simulink model "stm32f4_ds3231_configure_demo"  (Simulink 7.3)
settings: Solver=FixedStepDiscrete  SolverMode=SingleTasking  StartTime=0.0  StopTime=10.0  RelTol=1e-3
PreLoadFcn:
  | waijung.modelPreload; % Required for working with Waijung Blockset. Do not remove.
undefined symbols (not defined in the file): HSEOSC, Link, LQFP176, ST, STM32F417IG
libraries: simulink x94, amg_high_precision_rtc x5, stm32f4_io_lib x2, stm32f4_device_config_lib x1
(part 4 of 4)

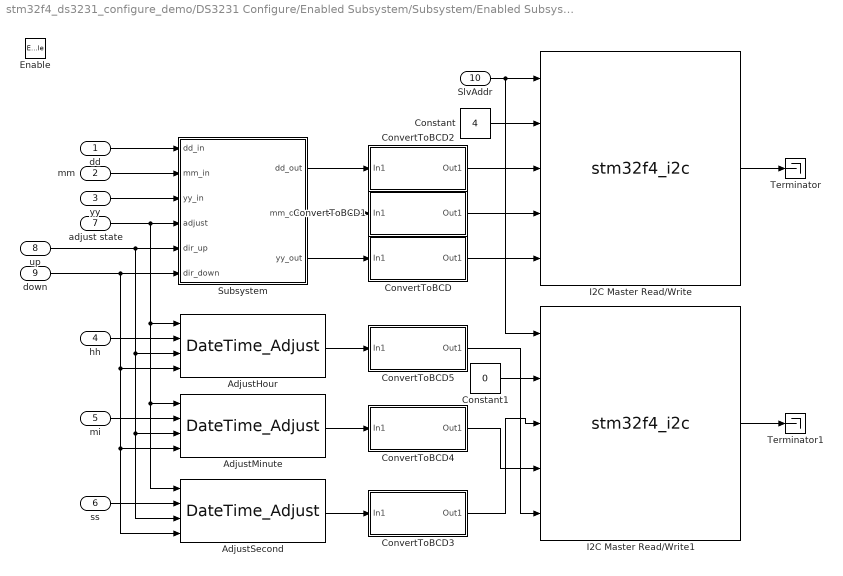
== system stm32f4_ds3231_configure_demo/DS3231 Configure/Enabled Subsystem/Subsystem/Enabled Subsystem ==
  dd : Inport  OutDataType=fixdt(1, 16)  OutScaling=2^0
  mm : Inport  Port=2  OutDataType=fixdt(1, 16)  OutScaling=2^0
  yy : Inport  Port=3  OutDataType=fixdt(1, 16)  OutScaling=2^0
  hh : Inport  Port=4  OutDataType=fixdt(1, 16)  OutScaling=2^0
  mi : Inport  Port=5  OutDataType=fixdt(1, 16)  OutScaling=2^0
  ss : Inport  Port=6  OutDataType=fixdt(1, 16)  OutScaling=2^0
  adjust state : Inport  Port=7  OutDataType=fixdt(1, 16)  OutScaling=2^0
  up : Inport  Port=8  OutDataType=fixdt(1, 16)  OutScaling=2^0
  down : Inport  Port=9  OutDataType=fixdt(1, 16)  OutScaling=2^0
  SlvAddr : Inport  Port=10  OutDataType=fixdt(1, 16)  OutScaling=2^0
  Enable : EnablePort
  AdjustHour : amg_high_precision_rtc/DateTime_Adjust  SystemSampleTime=-1  state=3  max=23  min=0
  AdjustMinute : amg_high_precision_rtc/DateTime_Adjust  SystemSampleTime=-1  state=4  max=59  min=0
  AdjustSecond : amg_high_precision_rtc/DateTime_Adjust  SystemSampleTime=-1  state=5  max=59  min=0
  Constant : Constant  Value=4  OutDataTypeMode=uint8  OutDataType=fixdt(1, 16)  OutScaling=2^0  OutDataTypeStr=uint8
  Constant1 : Constant  Value=0  OutDataTypeMode=uint8  OutDataType=fixdt(1, 16)  OutScaling=2^0  OutDataTypeStr=uint8
  ConvertToBCD : Subsystem  TreatAsAtomicUnit=on
      settings: RTWFcnNameOpts=Use subsystem name  RTWFileNameOpts=Use function name
      mask Display: disp('Dec-to-BCD');
  ConvertToBCD1 : Subsystem  TreatAsAtomicUnit=on
      settings: RTWFcnNameOpts=Use subsystem name  RTWFileNameOpts=Use function name
      mask Display: disp('Dec-to-BCD');
  ConvertToBCD2 : Subsystem  TreatAsAtomicUnit=on
      settings: RTWFcnNameOpts=Use subsystem name  RTWFileNameOpts=Use function name
      mask Display: disp('Dec-to-BCD');
  ConvertToBCD3 : Subsystem  TreatAsAtomicUnit=on
      settings: RTWFcnNameOpts=Use subsystem name  RTWFileNameOpts=Use function name
      mask Display: disp('Dec-to-BCD');
  ConvertToBCD4 : Subsystem  TreatAsAtomicUnit=on
      settings: RTWFcnNameOpts=Use subsystem name  RTWFileNameOpts=Use function name
      mask Display: disp('Dec-to-BCD');
  ConvertToBCD5 : Subsystem  TreatAsAtomicUnit=on
      settings: RTWFcnNameOpts=Use subsystem name  RTWFileNameOpts=Use function name
      mask Display: disp('Dec-to-BCD');
  I2C Master Read/Write : S-Function  FunctionName=stm32f4_i2c  Parameters=configuration,module,transfer,clkspeed,timeout,sdapin,sclpin,writecount,readcount,inputtypearray,outputtypearray,confstr,sampletime,sampletimestr,blockid  EnableBusSupport=off  mask(stm32f4_i2c){configuration=Transaction, module=1, lastmodule=3, transfer=Blocking, dutycycle=TLow/THigh = 2, clkspeed=400, timeout=25, writecount=4, readcount=0, sdapin=C9, sclpin=A8, waitwritetime=0, inputtypearray=[5 3 3 3 3 3], outputtypearray=[1 3], confstr=["C","9","A","8","1","1","6","0","I2C_DutyCycle_2","0","off"], sampletime=-1, sampletimestr=0.01, blockid=DS3231ConfigureEnabledSubsystemSubsystemEnabledSubsystemI2CMasterReadWrite}
      mask prompts: module "I2C Module"; lastmodule "Last module"; transfer "Transfer mode"; dutycycle "Duty cycle in fast mode"; clkspeed "Clock speed (kHz)"; timeout "Timeout (ms)"; writecount "Bytes write count"; readcount "Bytes read count"; sdapin "SDA pin"; sclpin "SCL pin"; waitwritetime "Wait write time (ms), default is 0"; inputtypearray "Input type array"; outputtypearray "Output type array"; confstr "Configuration string"; sampletime "Sample time (sec)"; sampletimestr "Compiled sample time (sec) in string"
      mask init:
      | stm32f4_i2c_callback('init');
      mask Help: web(fullfile(waijungdocroot,'stm32f4_i2c_readwrite.htm'), '-browser')
      mask StyleString: popup(Setup|Transaction),popup(1|2|3),edit,popup(Blocking|Non-blocking),popup(TLow/THigh = 16/9|TLow/THigh = 2),edit,edit,edit,edit,popup(-|C9),popup(-|A8),edit,edit,edit,edit,edit,edit,edit
      mask CallbackString: stm32f4_i2c_callback('configuration');|stm32f4_i2c_callback('module');|||stm32f4_i2c_callback('dutycycle');|||stm32f4_i2c_callback('writecount');|stm32f4_i2c_callback('readcount');|stm32f4_i2c_callback('sdapin');|stm32f4_i2c_callback('sclpin');||||stm32f4_i2c_callback('confstr');|stm32f4_i2c_callback('sampletime');|stm32f4_i2c_callback('sampletimestr');|stm32f4_i2c_callback('blockid');
      mask Display: text(0.5, 0.5, 'Module: I2C1\nTransfer: Blocking\nWrite: 4 bytes\nRead: 0 bytes\nTs (sec): 0.01','ver','middle','hor','center');port_label('input', 1,'SlvAddr');port_label('input', 2,'Wr0 (uint8)');port_label('input', 3,'Wr1 (uint8)');port_label('input', 4,'Wr2 (uint8)');port_label('input', 5,'Wr3 (uint8)');port_label('output', 1,'Status');
  I2C Master Read/Write1 : S-Function  FunctionName=stm32f4_i2c  Parameters=configuration,module,transfer,clkspeed,timeout,sdapin,sclpin,writecount,readcount,inputtypearray,outputtypearray,confstr,sampletime,sampletimestr,blockid  EnableBusSupport=off  mask(stm32f4_i2c){configuration=Transaction, module=1, lastmodule=3, transfer=Blocking, dutycycle=TLow/THigh = 2, clkspeed=400, timeout=25, writecount=4, readcount=0, sdapin=C9, sclpin=A8, waitwritetime=0, inputtypearray=[5 3 3 3 3 3], outputtypearray=[1 3], confstr=["C","9","A","8","1","1","6","0","I2C_DutyCycle_2","0","off"], sampletime=-1, sampletimestr=0.01, blockid=DS3231ConfigureEnabledSubsystemSubsystemEnabledSubsystemI2CMasterReadWrite1}
      mask prompts: module "I2C Module"; lastmodule "Last module"; transfer "Transfer mode"; dutycycle "Duty cycle in fast mode"; clkspeed "Clock speed (kHz)"; timeout "Timeout (ms)"; writecount "Bytes write count"; readcount "Bytes read count"; sdapin "SDA pin"; sclpin "SCL pin"; waitwritetime "Wait write time (ms), default is 0"; inputtypearray "Input type array"; outputtypearray "Output type array"; confstr "Configuration string"; sampletime "Sample time (sec)"; sampletimestr "Compiled sample time (sec) in string"
      mask init:
      | stm32f4_i2c_callback('init');
      mask Help: web(fullfile(waijungdocroot,'stm32f4_i2c_readwrite.htm'), '-browser')
      mask StyleString: popup(Setup|Transaction),popup(1|2|3),edit,popup(Blocking|Non-blocking),popup(TLow/THigh = 16/9|TLow/THigh = 2),edit,edit,edit,edit,popup(-|C9),popup(-|A8),edit,edit,edit,edit,edit,edit,edit
      mask CallbackString: stm32f4_i2c_callback('configuration');|stm32f4_i2c_callback('module');|||stm32f4_i2c_callback('dutycycle');|||stm32f4_i2c_callback('writecount');|stm32f4_i2c_callback('readcount');|stm32f4_i2c_callback('sdapin');|stm32f4_i2c_callback('sclpin');||||stm32f4_i2c_callback('confstr');|stm32f4_i2c_callback('sampletime');|stm32f4_i2c_callback('sampletimestr');|stm32f4_i2c_callback('blockid');
      mask Display: text(0.5, 0.5, 'Module: I2C1\nTransfer: Blocking\nWrite: 4 bytes\nRead: 0 bytes\nTs (sec): 0.01','ver','middle','hor','center');port_label('input', 1,'SlvAddr');port_label('input', 2,'Wr0 (uint8)');port_label('input', 3,'Wr1 (uint8)');port_label('input', 4,'Wr2 (uint8)');port_label('input', 5,'Wr3 (uint8)');port_label('output', 1,'Status');
  Subsystem : Subsystem
  Terminator : Terminator
  Terminator1 : Terminator
  wires:
  ConvertToBCD3/1(Out1) -> I2C Master Read/Write1/3
  ConvertToBCD5/1(Out1) -> I2C Master Read/Write1/5
  AdjustSecond/1 -> ConvertToBCD3/1(In1)
  AdjustMinute/1 -> ConvertToBCD4/1(In1)
  AdjustHour/1 -> ConvertToBCD5/1(In1)
  ConvertToBCD4/1(Out1) -> I2C Master Read/Write1/4
  I2C Master Read/Write1/1 -> Terminator1/1
  Constant1/1 -> I2C Master Read/Write1/2
  hh/1 -> AdjustHour/2
  mi/1 -> AdjustMinute/2
  ss/1 -> AdjustSecond/2
  ConvertToBCD/1(Out1) -> I2C Master Read/Write/5
  ConvertToBCD1/1(Out1) -> I2C Master Read/Write/4
  ConvertToBCD2/1(Out1) -> I2C Master Read/Write/3
  I2C Master Read/Write/1 -> Terminator/1
  Constant/1 -> I2C Master Read/Write/2
  Subsystem/3(yy_out) -> ConvertToBCD/1(In1)
  Subsystem/2(mm_out) -> ConvertToBCD1/1(In1)
  Subsystem/1(dd_out) -> ConvertToBCD2/1(In1)
  SlvAddr/1 -> I2C Master Read/Write1/1, I2C Master Read/Write/1
  down/1 -> AdjustSecond/4, AdjustMinute/4, AdjustHour/4, Subsystem/6(dir_down)
  up/1 -> AdjustSecond/3, AdjustMinute/3, AdjustHour/3, Subsystem/5(dir_up)
  adjust state/1 -> AdjustSecond/1, AdjustMinute/1, AdjustHour/1, Subsystem/4(adjust)
  yy/1 -> Subsystem/3(yy_in)
  mm/1 -> Subsystem/2(mm_in)
  dd/1 -> Subsystem/1(dd_in)

== system stm32f4_ds3231_configure_demo/Display Date/Time/Get Date as String/DS3231 Get Date/Convert ==
  In1 : Inport  OutDataType=fixdt(1, 16)  OutScaling=2^0
  In2 : Inport  Port=2  OutDataType=fixdt(1, 16)  OutScaling=2^0
  In3 : Inport  Port=3  OutDataType=fixdt(1, 16)  OutScaling=2^0
  In4 : Inport  Port=4  OutDataType=fixdt(1, 16)  OutScaling=2^0
  Enable : EnablePort
  Convert 1 : Subsystem
  Convert 2 : Subsystem
  Convert 3 : Subsystem
  Extract Bits : simulink/Logic and Bit Operations/Extract Bits  SystemSampleTime=-1  bitsToExtract=Range of bits  numBits=8  bitIdxRange=[0 3]  outScalingMode=Treat bit field as an integer
  Day : Outport  OutDataType=fixdt(1, 16)  OutScaling=2^0
  Date : Outport  Port=2  OutDataType=fixdt(1, 16)  OutScaling=2^0
  Month : Outport  Port=3  OutDataType=fixdt(1, 16)  OutScaling=2^0
  Year : Outport  Port=4  OutDataType=fixdt(1, 16)  OutScaling=2^0
  wires:
  Convert 3/1(Out1) -> Year/1
  In4/1 -> Convert 3/1(In1)
  Convert 2/1(Out1) -> Month/1
  In3/1 -> Convert 2/1(In1)
  In2/1 -> Convert 1/1(In1)
  Convert 1/1(Out1) -> Date/1
  Extract Bits/1 -> Day/1
  In1/1 -> Extract Bits/1

== system stm32f4_ds3231_configure_demo/Display Date/Time/Get Time as String/DS3231 Get Time/Convert ==
  In1 : Inport  OutDataType=fixdt(1, 16)  OutScaling=2^0
  In2 : Inport  Port=2  OutDataType=fixdt(1, 16)  OutScaling=2^0
  In3 : Inport  Port=3  OutDataType=fixdt(1, 16)  OutScaling=2^0
  Enable : EnablePort
  Convert Hour : Subsystem
  Convert Second/ Minute : Subsystem
  Demux : Demux  Outputs=2
  Mux : Mux  Inputs=2
  Hour : Outport  OutDataType=fixdt(1, 16)  OutScaling=2^0
  Minute : Outport  Port=2  OutDataType=fixdt(1, 16)  OutScaling=2^0
  Second : Outport  Port=3  OutDataType=fixdt(1, 16)  OutScaling=2^0
  AM/PM : Outport  Port=4  OutDataType=fixdt(1, 16)  OutScaling=2^0
  wires:
  Convert Hour/2(AM/PM) -> AM/PM/1
  Convert Hour/1(Hour) -> Hour/1
  In3/1 -> Convert Hour/1(In1)
  Demux/2 -> Minute/1
  Demux/1 -> Second/1
  Convert Second/ Minute/1(Out1) -> Demux/1
  Mux/1 -> Convert Second/ Minute/1(In1)
  In1/1 -> Mux/1
  In2/1 -> Mux/2

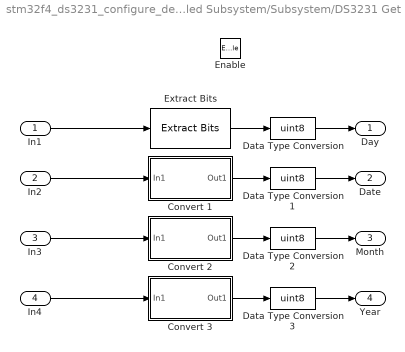
== system stm32f4_ds3231_configure_demo/DS3231 Configure/Enabled Subsystem/Subsystem/DS3231 Get Date/Convert ==
  In1 : Inport  OutDataType=fixdt(1, 16)  OutScaling=2^0
  In2 : Inport  Port=2  OutDataType=fixdt(1, 16)  OutScaling=2^0
  In3 : Inport  Port=3  OutDataType=fixdt(1, 16)  OutScaling=2^0
  In4 : Inport  Port=4  OutDataType=fixdt(1, 16)  OutScaling=2^0
  Enable : EnablePort
  Convert 1 : Subsystem
  Convert 2 : Subsystem
  Convert 3 : Subsystem
  Data Type Conversion{,1..3} (4 alike) : DataTypeConversion  OutDataTypeMode=uint8  OutDataType=fixdt(1, 16)  OutScaling=2^0  OutDataTypeStr=uint8
  Extract Bits : simulink/Logic and Bit Operations/Extract Bits  SystemSampleTime=-1  bitsToExtract=Range of bits  numBits=8  bitIdxRange=[0 3]  outScalingMode=Treat bit field as an integer
  Day : Outport  OutDataType=fixdt(1, 16)  OutScaling=2^0
  Date : Outport  Port=2  OutDataType=fixdt(1, 16)  OutScaling=2^0
  Month : Outport  Port=3  OutDataType=fixdt(1, 16)  OutScaling=2^0
  Year : Outport  Port=4  OutDataType=fixdt(1, 16)  OutScaling=2^0
  wires:
  In1/1 -> Extract Bits/1
  Extract Bits/1 -> Data Type Conversion/1
  Convert 1/1(Out1) -> Data Type Conversion1/1
  In2/1 -> Convert 1/1(In1)
  In3/1 -> Convert 2/1(In1)
  Convert 2/1(Out1) -> Data Type Conversion2/1
  In4/1 -> Convert 3/1(In1)
  Convert 3/1(Out1) -> Data Type Conversion3/1
  Data Type Conversion/1 -> Day/1
  Data Type Conversion1/1 -> Date/1
  Data Type Conversion2/1 -> Month/1
  Data Type Conversion3/1 -> Year/1

== system stm32f4_ds3231_configure_demo/DS3231 Configure/Enabled Subsystem/Subsystem/DS3231 Get Time/Convert ==
  In1 : Inport  OutDataType=fixdt(1, 16)  OutScaling=2^0
  In2 : Inport  Port=2  OutDataType=fixdt(1, 16)  OutScaling=2^0
  In3 : Inport  Port=3  OutDataType=fixdt(1, 16)  OutScaling=2^0
  Enable : EnablePort
  Convert Hour : Subsystem
  Convert Second/ Minute : Subsystem
  Demux : Demux  Outputs=2
  Mux : Mux  Inputs=2
  Hour : Outport  OutDataType=fixdt(1, 16)  OutScaling=2^0
  Minute : Outport  Port=2  OutDataType=fixdt(1, 16)  OutScaling=2^0
  Second : Outport  Port=3  OutDataType=fixdt(1, 16)  OutScaling=2^0
  AM/PM : Outport  Port=4  OutDataType=fixdt(1, 16)  OutScaling=2^0
  wires:
  In2/1 -> Mux/2
  In1/1 -> Mux/1
  Mux/1 -> Convert Second/ Minute/1(In1)
  Convert Second/ Minute/1(Out1) -> Demux/1
  Demux/1 -> Second/1
  Demux/2 -> Minute/1
  In3/1 -> Convert Hour/1(In1)
  Convert Hour/1(Hour) -> Hour/1
  Convert Hour/2(AM/PM) -> AM/PM/1

== system stm32f4_ds3231_configure_demo/DS3231 Configure/Enabled Subsystem/Subsystem/Enabled Subsystem/ConvertToBCD ==
  In1 : Inport  OutDataType=fixdt(1, 16)  OutScaling=2^0
  Bitwise Operator : simulink/Logic and Bit Operations/Bitwise Operator  logicop=OR  UseBitMask=off  NumInputPorts=2  BitMask=bin2dec('11011001')  BitMaskRealWorld=Stored Integer
  Constant : Constant  Value=10  OutDataTypeMode=single  OutDataType=fixdt(1, 16)  OutScaling=2^0  OutDataTypeStr=single
  Constant1 : Constant  Value=10  OutDataTypeMode=single  OutDataType=fixdt(1, 16)  OutScaling=2^0  OutDataTypeStr=single
  Data Type Conversion : DataTypeConversion  OutDataTypeMode=single  OutDataType=fixdt(1, 16)  OutScaling=2^0  OutDataTypeStr=single
  Data Type Conversion1 : DataTypeConversion  OutDataTypeMode=uint8  OutDataType=fixdt(1, 16)  OutScaling=2^0  OutDataTypeStr=uint8
  Data Type Conversion2 : DataTypeConversion  OutDataTypeMode=uint8  OutDataType=fixdt(1, 16)  OutScaling=2^0  OutDataTypeStr=uint8
  Data Type Conversion3 : DataTypeConversion  OutDataTypeMode=uint8  OutDataType=fixdt(1, 16)  OutScaling=2^0  OutDataTypeStr=uint8
  Divide : Product  Inputs=*/  OutDataType=fixdt(1, 16)  OutScaling=2^-10
  Product : Product  OutDataType=fixdt(1, 16)  OutScaling=2^0  RndMeth=Zero
  Shift Arithmetic : simulink/Logic and Bit Operations/Shift Arithmetic  SystemSampleTime=-1  nBitShiftRight=-4  nBinPtShiftRight=0
  Subtract : Sum  Inputs=+-  OutDataType=fixdt(1, 16)  OutScaling=2^-10
  Out1 : Outport  OutDataType=fixdt(1, 16)  OutScaling=2^0
  wires:
  Constant/1 -> Divide/2
  In1/1 -> Data Type Conversion/1, Subtract/1
  Data Type Conversion/1 -> Divide/1
  Divide/1 -> Data Type Conversion1/1
  Data Type Conversion1/1 -> Product/2, Shift Arithmetic/1
  Product/1 -> Subtract/2
  Constant1/1 -> Product/1
  Subtract/1 -> Data Type Conversion2/1
  Shift Arithmetic/1 -> Data Type Conversion3/1
  Data Type Conversion2/1 -> Bitwise Operator/1
  Data Type Conversion3/1 -> Bitwise Operator/2
  Bitwise Operator/1 -> Out1/1

== system stm32f4_ds3231_configure_demo/DS3231 Configure/Enabled Subsystem/Subsystem/Enabled Subsystem/ConvertToBCD1 ==
  In1 : Inport  OutDataType=fixdt(1, 16)  OutScaling=2^0
  Bitwise Operator : simulink/Logic and Bit Operations/Bitwise Operator  logicop=OR  UseBitMask=off  NumInputPorts=2  BitMask=bin2dec('11011001')  BitMaskRealWorld=Stored Integer
  Constant : Constant  Value=10  OutDataTypeMode=single  OutDataType=fixdt(1, 16)  OutScaling=2^0  OutDataTypeStr=single
  Constant1 : Constant  Value=10  OutDataTypeMode=single  OutDataType=fixdt(1, 16)  OutScaling=2^0  OutDataTypeStr=single
  Data Type Conversion : DataTypeConversion  OutDataTypeMode=single  OutDataType=fixdt(1, 16)  OutScaling=2^0  OutDataTypeStr=single
  Data Type Conversion1 : DataTypeConversion  OutDataTypeMode=uint8  OutDataType=fixdt(1, 16)  OutScaling=2^0  OutDataTypeStr=uint8
  Data Type Conversion2 : DataTypeConversion  OutDataTypeMode=uint8  OutDataType=fixdt(1, 16)  OutScaling=2^0  OutDataTypeStr=uint8
  Data Type Conversion3 : DataTypeConversion  OutDataTypeMode=uint8  OutDataType=fixdt(1, 16)  OutScaling=2^0  OutDataTypeStr=uint8
  Divide : Product  Inputs=*/  OutDataType=fixdt(1, 16)  OutScaling=2^-10
  Product : Product  OutDataType=fixdt(1, 16)  OutScaling=2^0  RndMeth=Zero
  Shift Arithmetic : simulink/Logic and Bit Operations/Shift Arithmetic  SystemSampleTime=-1  nBitShiftRight=-4  nBinPtShiftRight=0
  Subtract : Sum  Inputs=+-  OutDataType=fixdt(1, 16)  OutScaling=2^-10
  Out1 : Outport  OutDataType=fixdt(1, 16)  OutScaling=2^0
  wires:
  Constant/1 -> Divide/2
  In1/1 -> Data Type Conversion/1, Subtract/1
  Data Type Conversion/1 -> Divide/1
  Divide/1 -> Data Type Conversion1/1
  Data Type Conversion1/1 -> Product/2, Shift Arithmetic/1
  Product/1 -> Subtract/2
  Constant1/1 -> Product/1
  Subtract/1 -> Data Type Conversion2/1
  Shift Arithmetic/1 -> Data Type Conversion3/1
  Data Type Conversion2/1 -> Bitwise Operator/1
  Data Type Conversion3/1 -> Bitwise Operator/2
  Bitwise Operator/1 -> Out1/1

== system stm32f4_ds3231_configure_demo/DS3231 Configure/Enabled Subsystem/Subsystem/Enabled Subsystem/ConvertToBCD2 ==
  In1 : Inport  OutDataType=fixdt(1, 16)  OutScaling=2^0
  Bitwise Operator : simulink/Logic and Bit Operations/Bitwise Operator  logicop=OR  UseBitMask=off  NumInputPorts=2  BitMask=bin2dec('11011001')  BitMaskRealWorld=Stored Integer
  Constant : Constant  Value=10  OutDataTypeMode=single  OutDataType=fixdt(1, 16)  OutScaling=2^0  OutDataTypeStr=single
  Constant1 : Constant  Value=10  OutDataTypeMode=single  OutDataType=fixdt(1, 16)  OutScaling=2^0  OutDataTypeStr=single
  Data Type Conversion : DataTypeConversion  OutDataTypeMode=single  OutDataType=fixdt(1, 16)  OutScaling=2^0  OutDataTypeStr=single
  Data Type Conversion1 : DataTypeConversion  OutDataTypeMode=uint8  OutDataType=fixdt(1, 16)  OutScaling=2^0  OutDataTypeStr=uint8
  Data Type Conversion2 : DataTypeConversion  OutDataTypeMode=uint8  OutDataType=fixdt(1, 16)  OutScaling=2^0  OutDataTypeStr=uint8
  Data Type Conversion3 : DataTypeConversion  OutDataTypeMode=uint8  OutDataType=fixdt(1, 16)  OutScaling=2^0  OutDataTypeStr=uint8
  Divide : Product  Inputs=*/  OutDataType=fixdt(1, 16)  OutScaling=2^-10
  Product : Product  OutDataType=fixdt(1, 16)  OutScaling=2^0  RndMeth=Zero
  Shift Arithmetic : simulink/Logic and Bit Operations/Shift Arithmetic  SystemSampleTime=-1  nBitShiftRight=-4  nBinPtShiftRight=0
  Subtract : Sum  Inputs=+-  OutDataType=fixdt(1, 16)  OutScaling=2^-10
  Out1 : Outport  OutDataType=fixdt(1, 16)  OutScaling=2^0
  wires:
  Constant/1 -> Divide/2
  In1/1 -> Data Type Conversion/1, Subtract/1
  Data Type Conversion/1 -> Divide/1
  Divide/1 -> Data Type Conversion1/1
  Data Type Conversion1/1 -> Product/2, Shift Arithmetic/1
  Product/1 -> Subtract/2
  Constant1/1 -> Product/1
  Subtract/1 -> Data Type Conversion2/1
  Shift Arithmetic/1 -> Data Type Conversion3/1
  Data Type Conversion2/1 -> Bitwise Operator/1
  Data Type Conversion3/1 -> Bitwise Operator/2
  Bitwise Operator/1 -> Out1/1

== system stm32f4_ds3231_configure_demo/DS3231 Configure/Enabled Subsystem/Subsystem/Enabled Subsystem/ConvertToBCD3 ==
  In1 : Inport  OutDataType=fixdt(1, 16)  OutScaling=2^0
  Bitwise Operator : simulink/Logic and Bit Operations/Bitwise Operator  logicop=OR  UseBitMask=off  NumInputPorts=2  BitMask=bin2dec('11011001')  BitMaskRealWorld=Stored Integer
  Constant : Constant  Value=10  OutDataTypeMode=single  OutDataType=fixdt(1, 16)  OutScaling=2^0  OutDataTypeStr=single
  Constant1 : Constant  Value=10  OutDataTypeMode=single  OutDataType=fixdt(1, 16)  OutScaling=2^0  OutDataTypeStr=single
  Data Type Conversion : DataTypeConversion  OutDataTypeMode=single  OutDataType=fixdt(1, 16)  OutScaling=2^0  OutDataTypeStr=single
  Data Type Conversion1 : DataTypeConversion  OutDataTypeMode=uint8  OutDataType=fixdt(1, 16)  OutScaling=2^0  OutDataTypeStr=uint8
  Data Type Conversion2 : DataTypeConversion  OutDataTypeMode=uint8  OutDataType=fixdt(1, 16)  OutScaling=2^0  OutDataTypeStr=uint8
  Data Type Conversion3 : DataTypeConversion  OutDataTypeMode=uint8  OutDataType=fixdt(1, 16)  OutScaling=2^0  OutDataTypeStr=uint8
  Divide : Product  Inputs=*/  OutDataType=fixdt(1, 16)  OutScaling=2^-10
  Product : Product  OutDataType=fixdt(1, 16)  OutScaling=2^0  RndMeth=Zero
  Shift Arithmetic : simulink/Logic and Bit Operations/Shift Arithmetic  SystemSampleTime=-1  nBitShiftRight=-4  nBinPtShiftRight=0
  Subtract : Sum  Inputs=+-  OutDataType=fixdt(1, 16)  OutScaling=2^-10
  Out1 : Outport  OutDataType=fixdt(1, 16)  OutScaling=2^0
  wires:
  Constant/1 -> Divide/2
  In1/1 -> Data Type Conversion/1, Subtract/1
  Data Type Conversion/1 -> Divide/1
  Divide/1 -> Data Type Conversion1/1
  Data Type Conversion1/1 -> Product/2, Shift Arithmetic/1
  Product/1 -> Subtract/2
  Constant1/1 -> Product/1
  Subtract/1 -> Data Type Conversion2/1
  Shift Arithmetic/1 -> Data Type Conversion3/1
  Data Type Conversion2/1 -> Bitwise Operator/1
  Data Type Conversion3/1 -> Bitwise Operator/2
  Bitwise Operator/1 -> Out1/1

== system stm32f4_ds3231_configure_demo/DS3231 Configure/Enabled Subsystem/Subsystem/Enabled Subsystem/ConvertToBCD4 ==
  In1 : Inport  OutDataType=fixdt(1, 16)  OutScaling=2^0
  Bitwise Operator : simulink/Logic and Bit Operations/Bitwise Operator  logicop=OR  UseBitMask=off  NumInputPorts=2  BitMask=bin2dec('11011001')  BitMaskRealWorld=Stored Integer
  Constant : Constant  Value=10  OutDataTypeMode=single  OutDataType=fixdt(1, 16)  OutScaling=2^0  OutDataTypeStr=single
  Constant1 : Constant  Value=10  OutDataTypeMode=single  OutDataType=fixdt(1, 16)  OutScaling=2^0  OutDataTypeStr=single
  Data Type Conversion : DataTypeConversion  OutDataTypeMode=single  OutDataType=fixdt(1, 16)  OutScaling=2^0  OutDataTypeStr=single
  Data Type Conversion1 : DataTypeConversion  OutDataTypeMode=uint8  OutDataType=fixdt(1, 16)  OutScaling=2^0  OutDataTypeStr=uint8
  Data Type Conversion2 : DataTypeConversion  OutDataTypeMode=uint8  OutDataType=fixdt(1, 16)  OutScaling=2^0  OutDataTypeStr=uint8
  Data Type Conversion3 : DataTypeConversion  OutDataTypeMode=uint8  OutDataType=fixdt(1, 16)  OutScaling=2^0  OutDataTypeStr=uint8
  Divide : Product  Inputs=*/  OutDataType=fixdt(1, 16)  OutScaling=2^-10
  Product : Product  OutDataType=fixdt(1, 16)  OutScaling=2^0  RndMeth=Zero
  Shift Arithmetic : simulink/Logic and Bit Operations/Shift Arithmetic  SystemSampleTime=-1  nBitShiftRight=-4  nBinPtShiftRight=0
  Subtract : Sum  Inputs=+-  OutDataType=fixdt(1, 16)  OutScaling=2^-10
  Out1 : Outport  OutDataType=fixdt(1, 16)  OutScaling=2^0
  wires:
  Constant/1 -> Divide/2
  In1/1 -> Data Type Conversion/1, Subtract/1
  Data Type Conversion/1 -> Divide/1
  Divide/1 -> Data Type Conversion1/1
  Data Type Conversion1/1 -> Product/2, Shift Arithmetic/1
  Product/1 -> Subtract/2
  Constant1/1 -> Product/1
  Subtract/1 -> Data Type Conversion2/1
  Shift Arithmetic/1 -> Data Type Conversion3/1
  Data Type Conversion2/1 -> Bitwise Operator/1
  Data Type Conversion3/1 -> Bitwise Operator/2
  Bitwise Operator/1 -> Out1/1

== system stm32f4_ds3231_configure_demo/DS3231 Configure/Enabled Subsystem/Subsystem/Enabled Subsystem/ConvertToBCD5 ==
  In1 : Inport  OutDataType=fixdt(1, 16)  OutScaling=2^0
  Bitwise Operator : simulink/Logic and Bit Operations/Bitwise Operator  logicop=OR  UseBitMask=off  NumInputPorts=2  BitMask=bin2dec('11011001')  BitMaskRealWorld=Stored Integer
  Constant : Constant  Value=10  OutDataTypeMode=single  OutDataType=fixdt(1, 16)  OutScaling=2^0  OutDataTypeStr=single
  Constant1 : Constant  Value=10  OutDataTypeMode=single  OutDataType=fixdt(1, 16)  OutScaling=2^0  OutDataTypeStr=single
  Data Type Conversion : DataTypeConversion  OutDataTypeMode=single  OutDataType=fixdt(1, 16)  OutScaling=2^0  OutDataTypeStr=single
  Data Type Conversion1 : DataTypeConversion  OutDataTypeMode=uint8  OutDataType=fixdt(1, 16)  OutScaling=2^0  OutDataTypeStr=uint8
  Data Type Conversion2 : DataTypeConversion  OutDataTypeMode=uint8  OutDataType=fixdt(1, 16)  OutScaling=2^0  OutDataTypeStr=uint8
  Data Type Conversion3 : DataTypeConversion  OutDataTypeMode=uint8  OutDataType=fixdt(1, 16)  OutScaling=2^0  OutDataTypeStr=uint8
  Divide : Product  Inputs=*/  OutDataType=fixdt(1, 16)  OutScaling=2^-10
  Product : Product  OutDataType=fixdt(1, 16)  OutScaling=2^0  RndMeth=Zero
  Shift Arithmetic : simulink/Logic and Bit Operations/Shift Arithmetic  SystemSampleTime=-1  nBitShiftRight=-4  nBinPtShiftRight=0
  Subtract : Sum  Inputs=+-  OutDataType=fixdt(1, 16)  OutScaling=2^-10
  Out1 : Outport  OutDataType=fixdt(1, 16)  OutScaling=2^0
  wires:
  Constant/1 -> Divide/2
  In1/1 -> Data Type Conversion/1, Subtract/1
  Data Type Conversion/1 -> Divide/1
  Divide/1 -> Data Type Conversion1/1
  Data Type Conversion1/1 -> Product/2, Shift Arithmetic/1
  Product/1 -> Subtract/2
  Constant1/1 -> Product/1
  Subtract/1 -> Data Type Conversion2/1
  Shift Arithmetic/1 -> Data Type Conversion3/1
  Data Type Conversion2/1 -> Bitwise Operator/1
  Data Type Conversion3/1 -> Bitwise Operator/2
  Bitwise Operator/1 -> Out1/1

== system stm32f4_ds3231_configure_demo/DS3231 Configure/Enabled Subsystem/Subsystem/Enabled Subsystem/Subsystem ==
  dd_in : Inport  OutDataType=fixdt(1, 16)  OutScaling=2^0
  mm_in : Inport  Port=2  OutDataType=fixdt(1, 16)  OutScaling=2^0
  yy_in : Inport  Port=3  OutDataType=fixdt(1, 16)  OutScaling=2^0
  adjust : Inport  Port=4  OutDataType=fixdt(1, 16)  OutScaling=2^0
  dir_up : Inport  Port=5  OutDataType=fixdt(1, 16)  OutScaling=2^0
  dir_down : Inport  Port=6  OutDataType=fixdt(1, 16)  OutScaling=2^0
  AdjustMonth : amg_high_precision_rtc/DateTime_Adjust  SystemSampleTime=-1  state=1  max=12  min=1
  AdjustYear : amg_high_precision_rtc/DateTime_Adjust  SystemSampleTime=-1  state=2  max=99  min=0
  Day count : Subsystem
  Relational Operator : RelationalOperator  Operator=>  LogicOutDataTypeMode=boolean  LogicDataType=fixdt(0, 8)  OutDataTypeStr=boolean
  Subsystem : Subsystem
  Switch : Switch  Criteria=u2 ~= 0  OutDataType=fixdt(1, 16)  OutScaling=2^0
  dd_out : Outport  OutDataType=fixdt(1, 16)  OutScaling=2^0
  mm_out : Outport  Port=2  OutDataType=fixdt(1, 16)  OutScaling=2^0
  yy_out : Outport  Port=3  OutDataType=fixdt(1, 16)  OutScaling=2^0
  wires:
  Subsystem/1(Output) -> dd_out/1
  Relational Operator/1 -> Switch/2
  Day count/1(Day count of month) -> Subsystem/5(Day count), Switch/1, Relational Operator/2
  Switch/1 -> Subsystem/2(Input)
  dd_in/1 -> Switch/3, Relational Operator/1
  AdjustMonth/1 -> mm_out/1, Day count/1(Month)
  AdjustYear/1 -> yy_out/1, Day count/2(Year)
  mm_in/1 -> AdjustMonth/2
  yy_in/1 -> AdjustYear/2
  adjust/1 -> Subsystem/1(Function), AdjustMonth/1, AdjustYear/1
  dir_up/1 -> Subsystem/3(Up), AdjustMonth/3, AdjustYear/3
  dir_down/1 -> Subsystem/4(Down), AdjustMonth/4, AdjustYear/4

== system stm32f4_ds3231_configure_demo/Display Date/Time/Get Date as String/DS3231 Get Date/Convert/Convert 1 ==
  In1 : Inport
  Add : Sum  OutDataType=fixdt(1, 16)  OutScaling=2^-10
  Constant : Constant  Value=10  OutDataTypeMode=uint8  OutDataType=fixdt(1, 16)  OutScaling=2^0  OutDataTypeStr=uint8
  Extract Bits : simulink/Logic and Bit Operations/Extract Bits  SystemSampleTime=-1  bitsToExtract=Range of bits  numBits=8  bitIdxRange=[4 5]  outScalingMode=Treat bit field as an integer
  Extract Bits1 : simulink/Logic and Bit Operations/Extract Bits  SystemSampleTime=-1  bitsToExtract=Range of bits  numBits=8  bitIdxRange=[0 3]  outScalingMode=Treat bit field as an integer
  Product : Product  OutDataType=fixdt(1, 16)  OutScaling=2^0  RndMeth=Zero
  Out1 : Outport
  wires:
  Add/1 -> Out1/1
  Extract Bits1/1 -> Add/2
  Product/1 -> Add/1
  Extract Bits/1 -> Product/2
  Constant/1 -> Product/1
  In1/1 -> Extract Bits1/1, Extract Bits/1

== system stm32f4_ds3231_configure_demo/Display Date/Time/Get Date as String/DS3231 Get Date/Convert/Convert 2 ==
  In1 : Inport
  Add : Sum  OutDataType=fixdt(1, 16)  OutScaling=2^-10
  Constant : Constant  Value=10  OutDataTypeMode=uint8  OutDataType=fixdt(1, 16)  OutScaling=2^0  OutDataTypeStr=uint8
  Extract Bits : simulink/Logic and Bit Operations/Extract Bits  SystemSampleTime=-1  bitsToExtract=Range of bits  numBits=8  bitIdxRange=[4 4]  outScalingMode=Treat bit field as an integer
  Extract Bits1 : simulink/Logic and Bit Operations/Extract Bits  SystemSampleTime=-1  bitsToExtract=Range of bits  numBits=8  bitIdxRange=[0 3]  outScalingMode=Treat bit field as an integer
  Product : Product  OutDataType=fixdt(1, 16)  OutScaling=2^0  RndMeth=Zero
  Out1 : Outport
  wires:
  In1/1 -> Extract Bits/1, Extract Bits1/1
  Constant/1 -> Product/1
  Extract Bits/1 -> Product/2
  Product/1 -> Add/1
  Extract Bits1/1 -> Add/2
  Add/1 -> Out1/1

== system stm32f4_ds3231_configure_demo/Display Date/Time/Get Date as String/DS3231 Get Date/Convert/Convert 3 ==
  In1 : Inport
  Add : Sum  OutDataType=fixdt(1, 16)  OutScaling=2^-10
  Constant : Constant  Value=10  OutDataTypeMode=uint8  OutDataType=fixdt(1, 16)  OutScaling=2^0  OutDataTypeStr=uint8
  Extract Bits : simulink/Logic and Bit Operations/Extract Bits  SystemSampleTime=-1  bitsToExtract=Range of bits  numBits=8  bitIdxRange=[4 7]  outScalingMode=Treat bit field as an integer
  Extract Bits1 : simulink/Logic and Bit Operations/Extract Bits  SystemSampleTime=-1  bitsToExtract=Range of bits  numBits=8  bitIdxRange=[0 3]  outScalingMode=Treat bit field as an integer
  Product : Product  OutDataType=fixdt(1, 16)  OutScaling=2^0  RndMeth=Zero
  Out1 : Outport
  wires:
  Add/1 -> Out1/1
  Extract Bits1/1 -> Add/2
  Product/1 -> Add/1
  Extract Bits/1 -> Product/2
  Constant/1 -> Product/1
  In1/1 -> Extract Bits1/1, Extract Bits/1

== system stm32f4_ds3231_configure_demo/Display Date/Time/Get Time as String/DS3231 Get Time/Convert/Convert Hour ==
  In1 : Inport
  Add : Sum  OutDataType=fixdt(1, 16)  OutScaling=2^-10
  Constant : Constant  Value=10  OutDataTypeMode=uint8  OutDataType=fixdt(1, 16)  OutScaling=2^0  OutDataTypeStr=uint8
  Extract Bits : simulink/Logic and Bit Operations/Extract Bits  SystemSampleTime=-1  bitsToExtract=Range of bits  numBits=8  bitIdxRange=[4 5]  outScalingMode=Treat bit field as an integer
  Extract Bits1 : simulink/Logic and Bit Operations/Extract Bits  SystemSampleTime=-1  bitsToExtract=Range of bits  numBits=8  bitIdxRange=[0 3]  outScalingMode=Treat bit field as an integer
  Extract Bits2 : simulink/Logic and Bit Operations/Extract Bits  SystemSampleTime=-1  bitsToExtract=Range of bits  numBits=8  bitIdxRange=[5 5]  outScalingMode=Treat bit field as an integer
  Product : Product  OutDataType=fixdt(1, 16)  OutScaling=2^0  RndMeth=Zero
  Hour : Outport
  AM/PM : Outport  Port=2
  wires:
  Extract Bits2/1 -> AM/PM/1
  Extract Bits1/1 -> Add/2
  In1/1 -> Extract Bits2/1, Extract Bits1/1, Extract Bits/1
  Constant/1 -> Product/1
  Extract Bits/1 -> Product/2
  Product/1 -> Add/1
  Add/1 -> Hour/1

== system stm32f4_ds3231_configure_demo/Display Date/Time/Get Time as String/DS3231 Get Time/Convert/Convert Second/ Minute ==
  In1 : Inport
  Add : Sum  OutDataType=fixdt(1, 16)  OutScaling=2^-10
  Constant : Constant  Value=10  OutDataTypeMode=uint8  OutDataType=fixdt(1, 16)  OutScaling=2^0  OutDataTypeStr=uint8
  Extract Bits : simulink/Logic and Bit Operations/Extract Bits  SystemSampleTime=-1  bitsToExtract=Range of bits  numBits=8  bitIdxRange=[4 6]  outScalingMode=Treat bit field as an integer
  Extract Bits1 : simulink/Logic and Bit Operations/Extract Bits  SystemSampleTime=-1  bitsToExtract=Range of bits  numBits=8  bitIdxRange=[0 3]  outScalingMode=Treat bit field as an integer
  Product : Product  OutDataType=fixdt(1, 16)  OutScaling=2^0  RndMeth=Zero
  Out1 : Outport
  wires:
  Add/1 -> Out1/1
  Extract Bits1/1 -> Add/2
  Product/1 -> Add/1
  Extract Bits/1 -> Product/2
  Constant/1 -> Product/1
  In1/1 -> Extract Bits1/1, Extract Bits/1

== system stm32f4_ds3231_configure_demo/DS3231 Configure/Enabled Subsystem/Subsystem/DS3231 Get Date/Convert/Convert 1 ==
  In1 : Inport
  Add : Sum  OutDataType=fixdt(1, 16)  OutScaling=2^-10
  Constant : Constant  Value=10  OutDataTypeMode=uint8  OutDataType=fixdt(1, 16)  OutScaling=2^0  OutDataTypeStr=uint8
  Extract Bits : simulink/Logic and Bit Operations/Extract Bits  SystemSampleTime=-1  bitsToExtract=Range of bits  numBits=8  bitIdxRange=[4 5]  outScalingMode=Treat bit field as an integer
  Extract Bits1 : simulink/Logic and Bit Operations/Extract Bits  SystemSampleTime=-1  bitsToExtract=Range of bits  numBits=8  bitIdxRange=[0 3]  outScalingMode=Treat bit field as an integer
  Product : Product  OutDataType=fixdt(1, 16)  OutScaling=2^0  RndMeth=Zero
  Out1 : Outport
  wires:
  In1/1 -> Extract Bits/1, Extract Bits1/1
  Constant/1 -> Product/1
  Extract Bits/1 -> Product/2
  Product/1 -> Add/1
  Extract Bits1/1 -> Add/2
  Add/1 -> Out1/1

== system stm32f4_ds3231_configure_demo/DS3231 Configure/Enabled Subsystem/Subsystem/DS3231 Get Date/Convert/Convert 2 ==
  In1 : Inport
  Add : Sum  OutDataType=fixdt(1, 16)  OutScaling=2^-10
  Constant : Constant  Value=10  OutDataTypeMode=uint8  OutDataType=fixdt(1, 16)  OutScaling=2^0  OutDataTypeStr=uint8
  Extract Bits : simulink/Logic and Bit Operations/Extract Bits  SystemSampleTime=-1  bitsToExtract=Range of bits  numBits=8  bitIdxRange=[4 4]  outScalingMode=Treat bit field as an integer
  Extract Bits1 : simulink/Logic and Bit Operations/Extract Bits  SystemSampleTime=-1  bitsToExtract=Range of bits  numBits=8  bitIdxRange=[0 3]  outScalingMode=Treat bit field as an integer
  Product : Product  OutDataType=fixdt(1, 16)  OutScaling=2^0  RndMeth=Zero
  Out1 : Outport
  wires:
  Add/1 -> Out1/1
  Extract Bits1/1 -> Add/2
  Product/1 -> Add/1
  Extract Bits/1 -> Product/2
  Constant/1 -> Product/1
  In1/1 -> Extract Bits1/1, Extract Bits/1

== system stm32f4_ds3231_configure_demo/DS3231 Configure/Enabled Subsystem/Subsystem/DS3231 Get Date/Convert/Convert 3 ==
  In1 : Inport
  Add : Sum  OutDataType=fixdt(1, 16)  OutScaling=2^-10
  Constant : Constant  Value=10  OutDataTypeMode=uint8  OutDataType=fixdt(1, 16)  OutScaling=2^0  OutDataTypeStr=uint8
  Extract Bits : simulink/Logic and Bit Operations/Extract Bits  SystemSampleTime=-1  bitsToExtract=Range of bits  numBits=8  bitIdxRange=[4 7]  outScalingMode=Treat bit field as an integer
  Extract Bits1 : simulink/Logic and Bit Operations/Extract Bits  SystemSampleTime=-1  bitsToExtract=Range of bits  numBits=8  bitIdxRange=[0 3]  outScalingMode=Treat bit field as an integer
  Product : Product  OutDataType=fixdt(1, 16)  OutScaling=2^0  RndMeth=Zero
  Out1 : Outport
  wires:
  In1/1 -> Extract Bits/1, Extract Bits1/1
  Constant/1 -> Product/1
  Extract Bits/1 -> Product/2
  Product/1 -> Add/1
  Extract Bits1/1 -> Add/2
  Add/1 -> Out1/1

== system stm32f4_ds3231_configure_demo/DS3231 Configure/Enabled Subsystem/Subsystem/DS3231 Get Time/Convert/Convert Hour ==
  In1 : Inport
  Add : Sum  OutDataType=fixdt(1, 16)  OutScaling=2^-10
  Constant : Constant  Value=10  OutDataTypeMode=uint8  OutDataType=fixdt(1, 16)  OutScaling=2^0  OutDataTypeStr=uint8
  Extract Bits : simulink/Logic and Bit Operations/Extract Bits  SystemSampleTime=-1  bitsToExtract=Range of bits  numBits=8  bitIdxRange=[4 5]  outScalingMode=Treat bit field as an integer
  Extract Bits1 : simulink/Logic and Bit Operations/Extract Bits  SystemSampleTime=-1  bitsToExtract=Range of bits  numBits=8  bitIdxRange=[0 3]  outScalingMode=Treat bit field as an integer
  Extract Bits2 : simulink/Logic and Bit Operations/Extract Bits  SystemSampleTime=-1  bitsToExtract=Range of bits  numBits=8  bitIdxRange=[5 5]  outScalingMode=Treat bit field as an integer
  Product : Product  OutDataType=fixdt(1, 16)  OutScaling=2^0  RndMeth=Zero
  Hour : Outport
  AM/PM : Outport  Port=2
  wires:
  Add/1 -> Hour/1
  Product/1 -> Add/1
  Extract Bits/1 -> Product/2
  Constant/1 -> Product/1
  In1/1 -> Extract Bits/1, Extract Bits1/1, Extract Bits2/1
  Extract Bits1/1 -> Add/2
  Extract Bits2/1 -> AM/PM/1

== system stm32f4_ds3231_configure_demo/DS3231 Configure/Enabled Subsystem/Subsystem/DS3231 Get Time/Convert/Convert Second/ Minute ==
  In1 : Inport
  Add : Sum  OutDataType=fixdt(1, 16)  OutScaling=2^-10
  Constant : Constant  Value=10  OutDataTypeMode=uint8  OutDataType=fixdt(1, 16)  OutScaling=2^0  OutDataTypeStr=uint8
  Extract Bits : simulink/Logic and Bit Operations/Extract Bits  SystemSampleTime=-1  bitsToExtract=Range of bits  numBits=8  bitIdxRange=[4 6]  outScalingMode=Treat bit field as an integer
  Extract Bits1 : simulink/Logic and Bit Operations/Extract Bits  SystemSampleTime=-1  bitsToExtract=Range of bits  numBits=8  bitIdxRange=[0 3]  outScalingMode=Treat bit field as an integer
  Product : Product  OutDataType=fixdt(1, 16)  OutScaling=2^0  RndMeth=Zero
  Out1 : Outport
  wires:
  In1/1 -> Extract Bits/1, Extract Bits1/1
  Constant/1 -> Product/1
  Extract Bits/1 -> Product/2
  Product/1 -> Add/1
  Extract Bits1/1 -> Add/2
  Add/1 -> Out1/1

== system stm32f4_ds3231_configure_demo/DS3231 Configure/Enabled Subsystem/Subsystem/Enabled Subsystem/Subsystem/Day count ==
  Month : Inport  OutDataType=fixdt(1, 16)  OutScaling=2^0
  Year : Inport  Port=2  OutDataType=fixdt(1, 16)  OutScaling=2^0
  Constant : Constant  Value=30  OutDataTypeMode=uint8  OutDataType=fixdt(1, 16)  OutScaling=2^0  OutDataTypeStr=uint8
  Constant1 : Constant  Value=31  OutDataTypeMode=uint8  OutDataType=fixdt(1, 16)  OutScaling=2^0  OutDataTypeStr=uint8
  Days 30 : Subsystem
  Subsystem : Subsystem
  Switch : Switch  Criteria=u2 ~= 0  OutDataType=fixdt(1, 16)  OutScaling=2^0
  Switch1 : Switch  Criteria=u2 ~= 0  OutDataType=fixdt(1, 16)  OutScaling=2^0
  Day count of month : Outport  OutDataType=fixdt(1, 16)  OutScaling=2^0
  wires:
  Switch/1 -> Day count of month/1
  Switch1/1 -> Switch/3
  Constant1/1 -> Switch1/3
  Subsystem/2(Day count) -> Switch1/1
  Subsystem/1(Out1) -> Switch1/2
  Year/1 -> Subsystem/2(Year)
  Month/1 -> Subsystem/1(Month), Days 30/1(In1)
  Constant/1 -> Switch/1
  Days 30/1(Out1) -> Switch/2

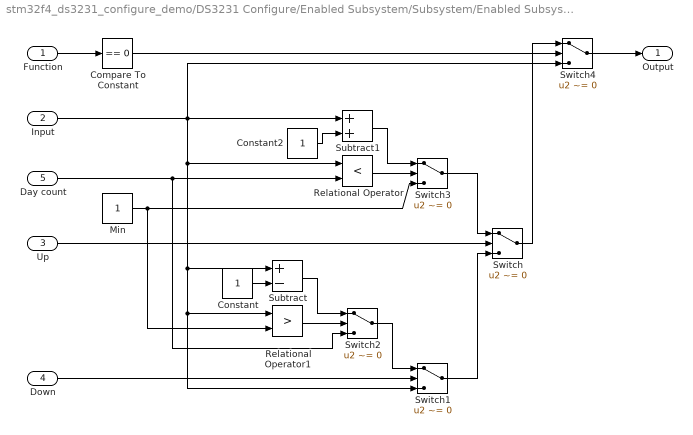
== system stm32f4_ds3231_configure_demo/DS3231 Configure/Enabled Subsystem/Subsystem/Enabled Subsystem/Subsystem/Subsystem ==
  Function : Inport  OutDataType=fixdt(1, 16)  OutScaling=2^0
  Input : Inport  Port=2  OutDataType=fixdt(1, 16)  OutScaling=2^0
  Up : Inport  Port=3  OutDataType=fixdt(1, 16)  OutScaling=2^0
  Down : Inport  Port=4  OutDataType=fixdt(1, 16)  OutScaling=2^0
  Day count : Inport  Port=5  OutDataType=fixdt(1, 16)  OutScaling=2^0
  Compare To Constant : simulink/Logic and Bit Operations/Compare To Constant  SystemSampleTime=-1  relop===  const=0  LogicOutDataTypeMode=uint8  ZeroCross=off
  Constant : Constant  OutDataTypeMode=uint8  OutDataType=fixdt(1, 16)  OutScaling=2^0  OutDataTypeStr=uint8
  Constant2 : Constant  OutDataTypeMode=uint8  OutDataType=fixdt(1, 16)  OutScaling=2^0  OutDataTypeStr=uint8
  Min : Constant  OutDataTypeMode=uint8  OutDataType=fixdt(1, 16)  OutScaling=2^0  OutDataTypeStr=uint8
  Relational Operator : RelationalOperator  Operator=<  LogicOutDataTypeMode=boolean  LogicDataType=fixdt(0, 8)  OutDataTypeStr=boolean
  Relational Operator1 : RelationalOperator  Operator=>  LogicOutDataTypeMode=boolean  LogicDataType=fixdt(0, 8)  OutDataTypeStr=boolean
  Subtract : Sum  Inputs=+-  OutDataType=fixdt(1, 16)  OutScaling=2^-10
  Subtract1 : Sum  OutDataType=fixdt(1, 16)  OutScaling=2^-10
  Switch{,1..4} (5 alike) : Switch  Criteria=u2 ~= 0  OutDataType=fixdt(1, 16)  OutScaling=2^0
  Output : Outport  OutDataType=fixdt(1, 16)  OutScaling=2^0
  wires:
  Up/1 -> Switch/2
  Down/1 -> Switch1/2
  Switch/1 -> Switch4/1
  Compare To Constant/1 -> Switch4/2
  Switch4/1 -> Output/1
  Function/1 -> Compare To Constant/1
  Switch3/1 -> Switch/1
  Day count/1 -> Switch2/3, Relational Operator/2
  Min/1 -> Relational Operator1/2, Switch3/3
  Constant2/1 -> Subtract1/2
  Subtract1/1 -> Switch3/1
  Relational Operator/1 -> Switch3/2
  Switch2/1 -> Switch1/1
  Constant/1 -> Subtract/2
  Subtract/1 -> Switch2/1
  Relational Operator1/1 -> Switch2/2
  Input/1 -> Switch4/3, Subtract1/1, Relational Operator/1, Relational Operator1/1, Switch1/3, Subtract/1
  Switch1/1 -> Switch/3

== system stm32f4_ds3231_configure_demo/DS3231 Configure/Enabled Subsystem/Subsystem/Enabled Subsystem/Subsystem/Day count/Days 30 ==
  In1 : Inport
  Bitwise Operator : simulink/Logic and Bit Operations/Bitwise Operator  logicop=OR  UseBitMask=off  NumInputPorts=4  BitMask=bin2dec('11011001')  BitMaskRealWorld=Stored Integer
  Compare To Constant : simulink/Logic and Bit Operations/Compare To Constant  SystemSampleTime=-1  relop===  const=6  LogicOutDataTypeMode=uint8  ZeroCross=off
  Compare To Constant1 : simulink/Logic and Bit Operations/Compare To Constant  SystemSampleTime=-1  relop===  const=4  LogicOutDataTypeMode=uint8  ZeroCross=off
  Compare To Constant2 : simulink/Logic and Bit Operations/Compare To Constant  SystemSampleTime=-1  relop===  const=9  LogicOutDataTypeMode=uint8  ZeroCross=off
  Compare To Constant3 : simulink/Logic and Bit Operations/Compare To Constant  SystemSampleTime=-1  relop===  const=11  LogicOutDataTypeMode=uint8  ZeroCross=off
  Out1 : Outport
  wires:
  Bitwise Operator/1 -> Out1/1
  In1/1 -> Compare To Constant3/1, Compare To Constant2/1, Compare To Constant/1, Compare To Constant1/1
  Compare To Constant3/1 -> Bitwise Operator/4
  Compare To Constant2/1 -> Bitwise Operator/3
  Compare To Constant/1 -> Bitwise Operator/2
  Compare To Constant1/1 -> Bitwise Operator/1

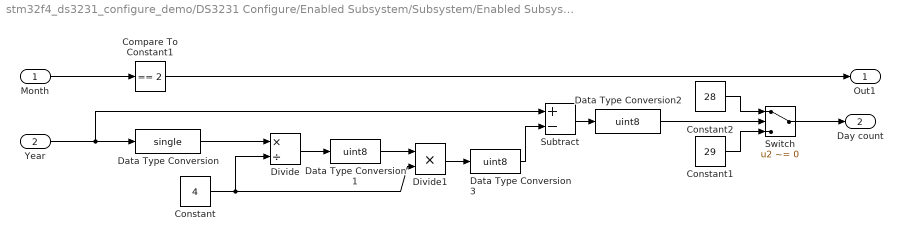
== system stm32f4_ds3231_configure_demo/DS3231 Configure/Enabled Subsystem/Subsystem/Enabled Subsystem/Subsystem/Day count/Subsystem ==
  Month : Inport  OutDataType=fixdt(1, 16)  OutScaling=2^0
  Year : Inport  Port=2  OutDataType=fixdt(1, 16)  OutScaling=2^0
  Compare To Constant1 : simulink/Logic and Bit Operations/Compare To Constant  SystemSampleTime=-1  relop===  const=2  LogicOutDataTypeMode=uint8  ZeroCross=off
  Constant : Constant  Value=4  OutDataTypeMode=single  OutDataType=fixdt(1, 16)  OutScaling=2^0  OutDataTypeStr=single
  Constant1 : Constant  Value=29  OutDataTypeMode=uint8  OutDataType=fixdt(1, 16)  OutScaling=2^0  OutDataTypeStr=uint8
  Constant2 : Constant  Value=28  OutDataTypeMode=uint8  OutDataType=fixdt(1, 16)  OutScaling=2^0  OutDataTypeStr=uint8
  Data Type Conversion : DataTypeConversion  OutDataTypeMode=single  OutDataType=fixdt(1, 16)  OutScaling=2^0  OutDataTypeStr=single
  Data Type Conversion1 : DataTypeConversion  OutDataTypeMode=uint8  OutDataType=fixdt(1, 16)  OutScaling=2^0  OutDataTypeStr=uint8
  Data Type Conversion2 : DataTypeConversion  OutDataTypeMode=uint8  OutDataType=fixdt(1, 16)  OutScaling=2^0  OutDataTypeStr=uint8
  Data Type Conversion3 : DataTypeConversion  OutDataTypeMode=uint8  OutDataType=fixdt(1, 16)  OutScaling=2^0  OutDataTypeStr=uint8
  Divide : Product  Inputs=*/  OutDataType=fixdt(1, 16)  OutScaling=2^-10
  Divide1 : Product  Inputs=**  OutDataType=fixdt(1, 16)  OutScaling=2^-10
  Subtract : Sum  Inputs=+-  OutDataType=fixdt(1, 16)  OutScaling=2^-10
  Switch : Switch  Criteria=u2 ~= 0  OutDataType=fixdt(1, 16)  OutScaling=2^0
  Out1 : Outport  OutDataType=fixdt(1, 16)  OutScaling=2^0
  Day count : Outport  Port=2  OutDataType=fixdt(1, 16)  OutScaling=2^0
  wires:
  Data Type Conversion3/1 -> Subtract/2
  Divide1/1 -> Data Type Conversion3/1
  Data Type Conversion1/1 -> Divide1/1
  Data Type Conversion2/1 -> Switch/2
  Switch/1 -> Day count/1
  Constant2/1 -> Switch/1
  Constant1/1 -> Switch/3
  Subtract/1 -> Data Type Conversion2/1
  Divide/1 -> Data Type Conversion1/1
  Constant/1 -> Divide1/2, Divide/2
  Data Type Conversion/1 -> Divide/1
  Year/1 -> Subtract/1, Data Type Conversion/1
  Compare To Constant1/1 -> Out1/1
  Month/1 -> Compare To Constant1/1
